simulink model "ConfrontoRispostaDelGradino"  (R2022b)
settings: Solver=VariableStepAuto  StartTime=0.0  StopTime=50  RelTol=1e-3
values from neighbouring files (symbols this model uses):
  c = c1(1,j)    [MassaMolla.m]
  h = 1.1    [Facoltativo.m]    (also in MassaMolla.m; MassaMollaLineare.m)
  k = 0.33    [Facoltativo.m]    (also in MassaMolla.m; MassaMollaLineare.m)
  M = 1.0    (= 1)    [Facoltativo.m]    (also in MassaMolla.m; MassaMollaLineare.m)
  x0 = x(i,:)'    [MassaMolla.m]
undefined symbols (not defined in the file or in its folder): Al, Bl, Cl, Dl, U, Y
settings Model: LastModifiedBy=TAWADROS
settings OptimizationCC: BlockReduction=off  BooleanDataType=off
settings DebuggingCC: SaveWithParameterizedLinksMsg=none  UnderspecifiedInitializationDetection=Classic  MergeDetectMultiDrivingBlocksExec=none  SignalResolutionControl=TryResolveAllWithWarning
settings HardwareCC: TargetUnknown=on
settings ModelReferenceCC: PropagateSignalLabelsOutOfModel=off

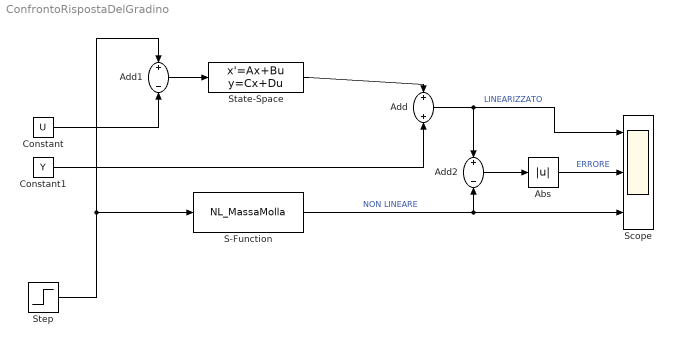
== system ConfrontoRispostaDelGradino ==
  Abs : Abs  SaturateOnIntegerOverflow=off
  Add : Sum
  Add1 : Sum  Inputs=+-
  Add2 : Sum  Inputs=+-
  Constant : Constant  Value=U
  Constant1 : Constant  Value=Y
  S-Function : S-Function  FunctionName=NL_MassaMolla  Parameters=M,k,h,x0  SFunctionDeploymentMode=off  EnableBusSupport=off
  Scope : Scope  NumInputPorts=3
  State-Space : StateSpace  A=Al  B=Bl  C=Cl  D=Dl  InitialCondition=0  ParameterTunability=Optimized
  Step : Step  Time=5  Before=U  After=c*U  SampleTime=2  VectorParams1D=off  ZeroCross=off
  wires:
  Add/1 -> Scope/1, Add2/1  "LINEARIZZATO"
  Add1/1 -> State-Space/1
  State-Space/1 -> Add/1
  Constant1/1 -> Add/2
  Constant/1 -> Add1/2
  S-Function/1 -> Scope/3, Add2/2  "NON LINEARE"
  Add2/1 -> Abs/1
  Step/1 -> S-Function/1, Add1/1
  Abs/1 -> Scope/2  "ERRORE"
